simulink model "bengji"  (R2021a)
settings: Solver=FixedStepAuto  StartTime=0.0  StopTime=50.0  FixedStep=0.1  RelTol=1e-3
model workspace (MAT data in the model file):
  times = 1
settings Model: Creator=86137  LastModifiedBy=86137

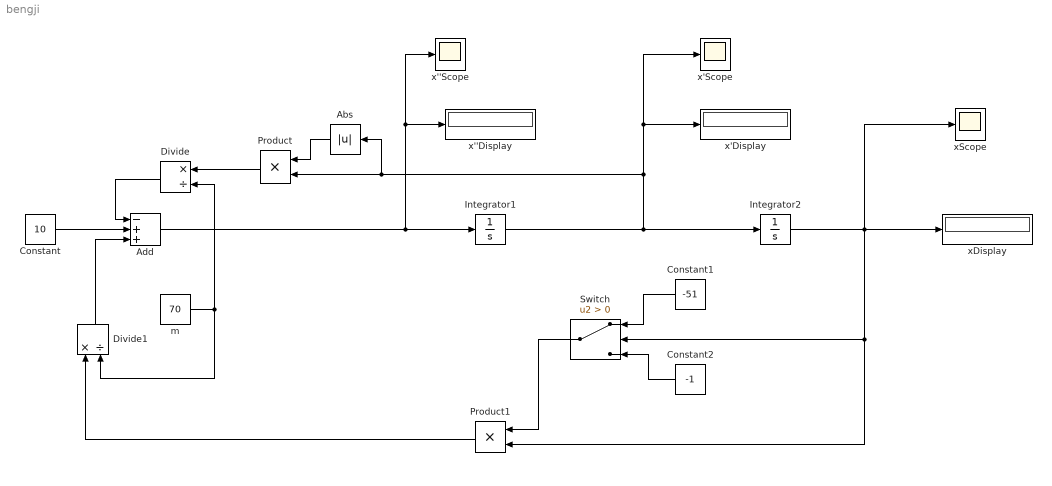
== system bengji ==
  Abs : Abs
  Add : Sum  Inputs=-++
  Constant : Constant  Value=10
  Constant1 : Constant  Value=-51
  Constant2 : Constant  Value=-1
  Divide : Product  Inputs=*/
  Divide1 : Product  Inputs=*/
  Integrator1 : Integrator
  Integrator2 : Integrator  InitialCondition=-30
  Product : Product
  Product1 : Product
  Switch : Switch  Criteria=u2 > Threshold
  m : Constant  Value=70
  x''Display : Display
  x''Scope : Scope
  x'Display : Display
  x'Scope : Scope
  xDisplay : Display
  xScope : Scope
  wires:
  Constant/1 -> Add/2
  Add/1 -> x''Display/1, x''Scope/1, Integrator1/1
  Integrator1/1 -> x'Display/1, x'Scope/1, Abs/1, Product/2, Integrator2/1
  Abs/1 -> Product/1
  Product/1 -> Divide/1
  Divide/1 -> Add/1
  m/1 -> Divide1/2, Divide/2
  Integrator2/1 -> Switch/2, Product1/2, xScope/1, xDisplay/1
  Divide1/1 -> Add/3
  Constant2/1 -> Switch/3
  Constant1/1 -> Switch/1
  Switch/1 -> Product1/1
  Product1/1 -> Divide1/1
